simulink model "MRACimple"  (R2022a)
settings: Solver=FixedStepAuto  StartTime=0.0  StopTime=inf  FixedStep=0.0001  RelTol=1e-3
undefined symbols (not defined in the file): a, a_m, b, b_m, c
settings Model: Creator=edgar  LastModifiedBy=edgar

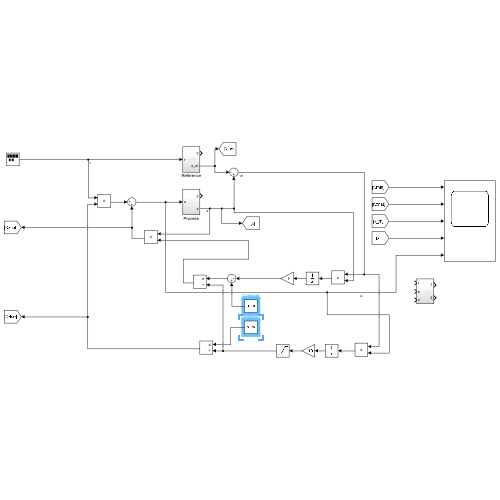
[thumbnail: Simulink's stored preview of the top-level diagram]
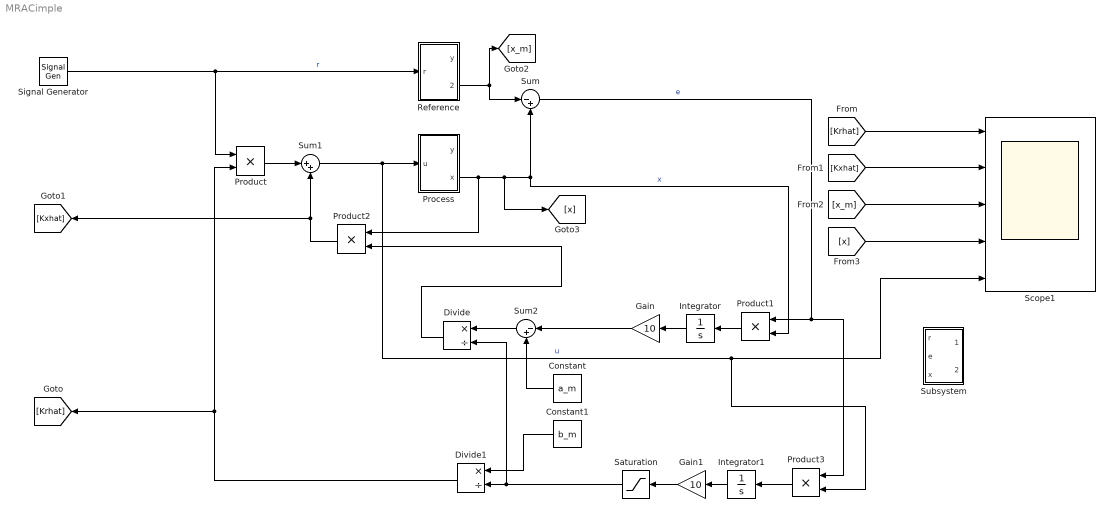
== system MRACimple ==
  Constant : Constant  Value=a_m
  Constant1 : Constant  Value=b_m
  Divide : Product  Inputs=*/
  Divide1 : Product  Inputs=*/
  Gain : Gain  Gain=10
  Gain1 : Gain  Gain=10
  Integrator : Integrator  InitialCondition=1
  Integrator1 : Integrator  InitialCondition=1
  Process : Subsystem
  Product{,1..3} (4 alike) : Product
  Reference : Subsystem
  Saturation : Saturate  UpperLimit=1000  LowerLimit=0.1
  Scope1 : Scope  NumInputPorts=5
  Signal Generator : SignalGenerator  WaveForm=square  Frequency=0.2  Units=rad/sec
  Subsystem : Subsystem
  Sum : Sum  Inputs=|-+
  Sum1 : Sum  Inputs=|++
  Sum2 : Sum  Inputs=|-+
  wires:
  [Kxhat] -> Scope1/2
  [x_m] -> Scope1/3
  Product2/1 -> [Kxhat], Sum1/2
  [x] -> Scope1/4
  Reference/2(x_m) -> [x_m], Sum/1
  [Krhat] -> Scope1/1
  Product/1 -> Sum1/1
  Process/2(x) -> Product2/1, Product1/2, Sum/2, [x]  "x"
  Sum1/1 -> Scope1/5, Product3/2, Process/1(u)  "u"
  Signal Generator/1 -> Reference/1(r), Product/1  "r"
  Sum/1 -> Product1/1, Product3/1  "e"
  Product1/1 -> Integrator/1
  Integrator/1 -> Gain/1
  Gain/1 -> Sum2/1
  Constant/1 -> Sum2/2
  Sum2/1 -> Divide/1
  Constant1/1 -> Divide1/1
  Divide/1 -> Product2/2
  Product3/1 -> Integrator1/1
  Integrator1/1 -> Gain1/1
  Divide1/1 -> [Krhat], Product/2
  Gain1/1 -> Saturation/1
  Saturation/1 -> Divide/2, Divide1/2

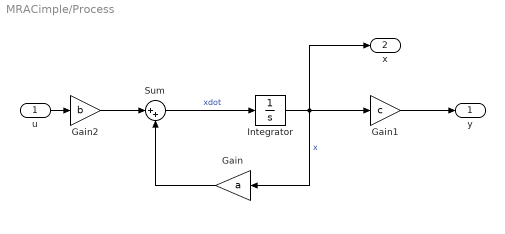
== system MRACimple/Process ==
  u : Inport
  Gain : Gain  Gain=a
  Gain1 : Gain  Gain=c
  Gain2 : Gain  Gain=b
  Integrator : Integrator
  Sum : Sum  Inputs=|++
  y : Outport
  x : Outport  Port=2
  wires:
  Sum/1 -> Integrator/1  "xdot"
  Integrator/1 -> x/1, Gain1/1, Gain/1  "x"
  Gain1/1 -> y/1
  Gain2/1 -> Sum/1
  Gain/1 -> Sum/2
  u/1 -> Gain2/1

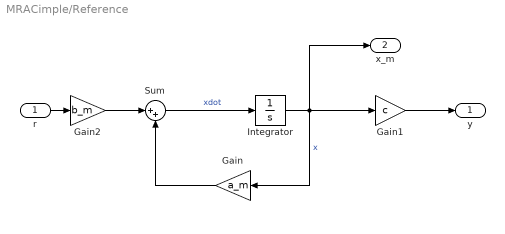
== system MRACimple/Reference ==
  r : Inport
  Gain : Gain  Gain=a_m
  Gain1 : Gain  Gain=c
  Gain2 : Gain  Gain=b_m
  Integrator : Integrator
  Sum : Sum  Inputs=|++
  y : Outport
  x_m : Outport  Port=2
  wires:
  Sum/1 -> Integrator/1  "xdot"
  Integrator/1 -> x_m/1, Gain1/1, Gain/1  "x"
  Gain1/1 -> y/1
  Gain2/1 -> Sum/1
  Gain/1 -> Sum/2
  r/1 -> Gain2/1

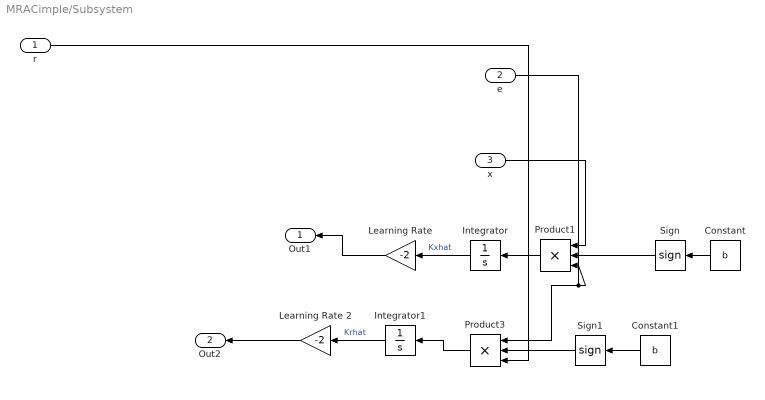
== system MRACimple/Subsystem ==
  r : Inport
  e : Inport  Port=2
  x : Inport  Port=3
  Constant : Constant  Value=b
  Constant1 : Constant  Value=b
  Integrator : Integrator
  Integrator1 : Integrator
  Learning Rate : Gain  Gain=-2
  "Learning Rate 2 " : Gain  Gain=-2
  Product1 : Product  Inputs=3
  Product3 : Product  Inputs=3
  Sign : Signum
  Sign1 : Signum
  Out1 : Outport
  Out2 : Outport  Port=2
  wires:
  Product1/1 -> Integrator/1
  Integrator1/1 -> "Learning Rate 2 "/1  "Krhat"
  r/1 -> Product3/3
  e/1 -> Product1/3, Product3/1
  Product3/1 -> Integrator1/1
  Constant/1 -> Sign/1
  Sign/1 -> Product1/2
  Integrator/1 -> Learning Rate/1  "Kxhat"
  Sign1/1 -> Product3/2
  "Learning Rate 2 "/1 -> Out2/1
  Constant1/1 -> Sign1/1
  Learning Rate/1 -> Out1/1
  x/1 -> Product1/1
